simulink model "Part5_workingSpace"  (R2018a)
settings: Solver=VariableStepAuto  StartTime=0.0  StopTime=2  RelTol=1e-3
values from neighbouring files (symbols this model uses):
  qqs = [t' qq]    [trajCircle.m]    (also in trajLine.m)
libraries: roblocks x3, simulink x1, dspmathops x1
settings Model: Creator=Francesco  LastModifiedBy=Francesco

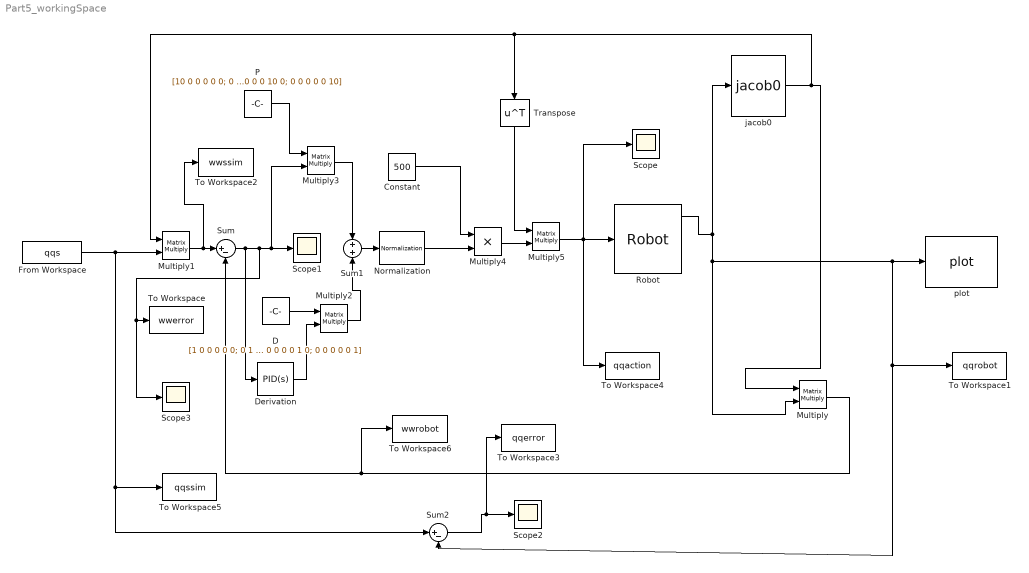
== system Part5_workingSpace ==
  Constant : Constant  Value=500
  D : Constant  Value=[1 0 0 0 0 0; 0 1 0 0 0 0; 0 0 1 0 0 0; 0 0 0 1 0 0; 0 0 0 0 1 0; 0 0 0 0 0 1]
  "Derivation " : simulink/Continuous/PID Controller  Controller=PID  TimeDomain=Continuous-time  SampleTime=-1  IntegratorMethod=Forward Euler  FilterMethod=Forward Euler  Form=Parallel  UseFilter=on  ControllerParametersSource=internal  P=0  I=0  D=1  N=100  InitialConditionSource=internal  InitialConditionForIntegrator=0  InitialConditionForFilter=0  ExternalReset=none  LimitOutput=off  UpperSaturationLimit=inf  LowerSaturationLimit=-inf  LinearizeAsGain=on  AntiWindupMode=none  Kb=1  TrackingMode=off  Kt=1  PParamMin=[]  PParamMax=[]  IParamMin=[]  IParamMax=[]  DParamMin=[]  DParamMax=[]  NParamMin=[]  NParamMax=[]  KbParamMin=[]  KbParamMax=[]  KtParamMin=[]  KtParamMax=[]  POutMin=[]  POutMax=[]  IOutMin=[]  IOutMax=[]  DOutMin=[]  DOutMax=[]  NOutMin=[]  NOutMax=[]  KbOutMin=[]  KbOutMax=[]  KtOutMin=[]  KtOutMax=[]  IntegratorOutMin=[]  IntegratorOutMax=[]  FilterOutMin=[]  FilterOutMax=[]  SumOutMin=[]  SumOutMax=[]  SumI1OutMin=[]  SumI1OutMax=[]  SumI2OutMin=[]  SumI2OutMax=[]  SumI3OutMin=[]  SumI3OutMax=[]  SumDOutMin=[]  SumDOutMax=[]  SaturationOutMin=[]  SaturationOutMax=[]  IntegratorContinuousStateAttributes=''  IntegratorStateMustResolveToSignalObject=off  IntegratorRTWStateStorageClass=Auto  FilterContinuousStateAttributes=''  FilterStateMustResolveToSignalObject=off  FilterRTWStateStorageClass=Auto  DifferentiatorICPrevScaledInput=0  DifferentiatorOutMin=[]  DifferentiatorOutMax=[]  FilterDiffOutCoefMin=[]  FilterDiffOutCoefMax=[]  SumDenOutMin=[]  SumDenOutMax=[]  SumNumOutMin=[]  SumNumOutMax=[]  ReciprocalOutMin=[]  ReciprocalOutMax=[]  DivideOutMin=[]  DivideOutMax=[]  TunerSelectOption=Transfer Function Based (PID Tuner App)
  From Workspace : FromWorkspace  VariableName=qqs  SampleTime=0
  Multiply{,1..3,5} (5 alike) : Product  Multiplication=Matrix(*)
  Multiply4 : Product
  Normalization : dspmathops/Normalization  NormType=2-norm  Bias=1e-10  NormOver=Each column  Dimension=1  roundingMode=Floor  overflowMode=off  accumDataTypeStr=Inherit: Same as product output  accumLastDataTypeStr=Inherit: Same as product output  outputDataTypeStr=Inherit: Same as product output  outputMin=[]  outputMax=[]  outputLastDataTypeStr=Inherit: Same as product output
      settings: SourceProductName=DSP System Toolbox
  P : Constant  Value=[10 0 0 0 0 0; 0 10 0 0 0 0; 0 0 10 0 0 0; 0 0 0 10 0 0; 0 0 0 0 10 0; 0 0 0 0 0 10]
  Robot : roblocks/Arm/Robot  robot=pumanofriction  q0=qqs(1, 2:7) + [0.1 0.1 0.1 0.1 0.1 0.1]
  Scope{,1..3} (4 alike) : Scope
  Sum : Sum  Inputs=|+-
  Sum1 : Sum
  Sum2 : Sum  Inputs=|+-
  To Workspace : ToWorkspace  VariableName=wwerror  SaveFormat=Structure With Time  SampleTime=-1
  To Workspace1 : ToWorkspace  VariableName=qqrobot  SaveFormat=Structure With Time  SampleTime=-1
  To Workspace2 : ToWorkspace  VariableName=wwssim  SaveFormat=Structure With Time  SampleTime=-1
  To Workspace3 : ToWorkspace  VariableName=qqerror  SaveFormat=Structure With Time  SampleTime=-1
  To Workspace4 : ToWorkspace  VariableName=qqaction  SaveFormat=Structure With Time  SampleTime=-1
  To Workspace5 : ToWorkspace  VariableName=qqssim  SaveFormat=Structure With Time  SampleTime=-1
  To Workspace6 : ToWorkspace  VariableName=wwrobot  SaveFormat=Structure With Time  SampleTime=-1
  Transpose : Math  Operator=transpose  SaturateOnIntegerOverflow=on
  "jacob0 " : roblocks/Arm/jacob0   robot=pumanofriction
  plot : roblocks/Arm/plot  robot=pumanofriction  fps=5  holdplot=on
  wires:
  Robot/1 -> Multiply/2, To Workspace1/1, Sum2/2, plot/1, "jacob0 "/1
  "jacob0 "/1 -> Transpose/1, Multiply1/1, Multiply/1
  Multiply/1 -> To Workspace6/1, Sum/2
  Multiply1/1 -> To Workspace2/1, Sum/1
  Sum/1 -> "Derivation "/1, Scope3/1, To Workspace/1, Scope1/1, Multiply3/2
  "Derivation "/1 -> Multiply2/2
  D/1 -> Multiply2/1
  P/1 -> Multiply3/1
  Multiply2/1 -> Sum1/2
  Multiply3/1 -> Sum1/1
  Sum1/1 -> Normalization/1
  Normalization/1 -> Multiply4/2
  Constant/1 -> Multiply4/1
  Multiply5/1 -> To Workspace4/1, Scope/1, Robot/1
  Transpose/1 -> Multiply5/1
  Multiply4/1 -> Multiply5/2
  Sum2/1 -> To Workspace3/1, Scope2/1
  From Workspace/1 -> To Workspace5/1, Sum2/1, Multiply1/2
